simulink model "firstcontroller"  (R2021b)
settings: Solver=VariableStepAuto  StartTime=0.0  StopTime=10  RelTol=1e-3
libraries: dspsrcs4 x1
settings Model: Creator=Asus  LastModifiedBy=Matina Kaviani
settings SolverCC: AlgebraicLoopSolver=TrustRegion
settings DebuggingCC: SFMachineParentedDataDiag=warning

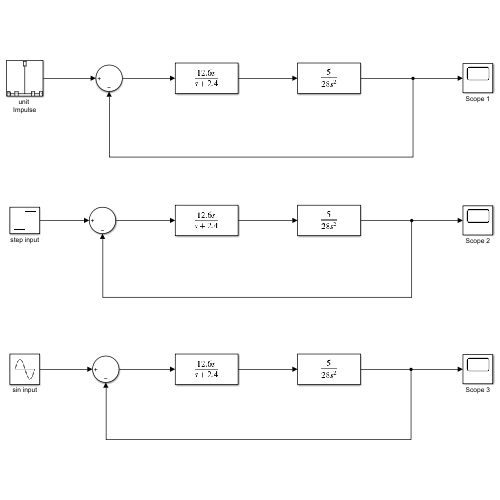
[thumbnail: Simulink's stored preview of the top-level diagram]
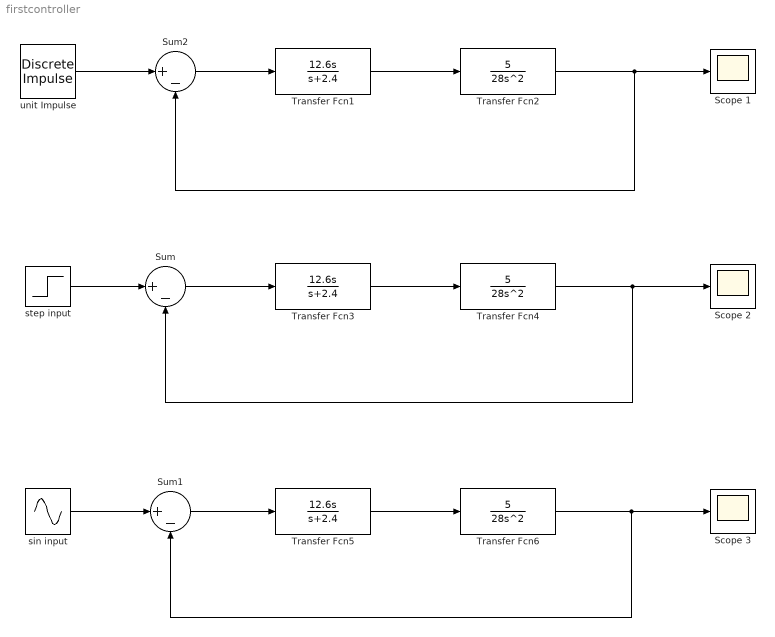
== system firstcontroller ==
  Scope 1 : Scope
  Scope 2 : Scope
  Scope 3 : Scope
  Sum : Sum  Inputs=|+-
  Sum1 : Sum  Inputs=|+-
  Sum2 : Sum  Inputs=|+-
  Transfer Fcn1 : TransferFcn  Numerator=[12.6 0]  Denominator=[1 2.4]
  Transfer Fcn2 : TransferFcn  Numerator=[0 5]  Denominator=[28 0 0]
  Transfer Fcn3 : TransferFcn  Numerator=[12.6 0]  Denominator=[1 2.4]
  Transfer Fcn4 : TransferFcn  Numerator=[0 5]  Denominator=[28 0 0]
  Transfer Fcn5 : TransferFcn  Numerator=[12.6 0]  Denominator=[1 2.4]
  Transfer Fcn6 : TransferFcn  Numerator=[0 5]  Denominator=[28 0 0]
  sin input : Sin  Frequency=2*pi  SampleTime=0
  step input : Step  After=2  SampleTime=0
  unit Impulse : dspsrcs4/Discrete  Impulse  Delay=0  SampleTime=1  FrameSample=1  OutputFrames=off  dataType=double  isSigned=on  wordLen=16  udDataType=sfix(16)  fracBitsMode=Best precision  numFracBits=15  OutDataTypeStr=double  LastOutDataTypeStr=double
  wires:
  Transfer Fcn3/1 -> Transfer Fcn4/1
  step input/1 -> Sum/1
  Sum/1 -> Transfer Fcn3/1
  Transfer Fcn4/1 -> Sum/2, Scope 2/1
  Transfer Fcn5/1 -> Transfer Fcn6/1
  Transfer Fcn6/1 -> Sum1/2, Scope 3/1
  sin input/1 -> Sum1/1
  Sum1/1 -> Transfer Fcn5/1
  unit Impulse/1 -> Sum2/1
  Sum2/1 -> Transfer Fcn1/1
  Transfer Fcn1/1 -> Transfer Fcn2/1
  Transfer Fcn2/1 -> Sum2/2, Scope 1/1
